simulink model "c63_cylinder_adiabatic_ref"  (R2026a)
settings: Solver=FixedStepDiscrete  StopTime=0  FixedStep=1e-4
model workspace (MAT data in the model file):
  S12_C63_BoreM = Simulink.Parameter
  S12_C63_BoreM.Value = 0.1022
  S12_C63_BoreM.Complexity = 'real'
  S12_C63_BoreM.Dimensions = [1 1]
  S12_C63_BoreM.Description = 'Grade A: Mercedes-Benz Public Archive M156.985 bore'
  S12_C63_BoreM.DataType = 'auto'
  S12_C63_BoreM.DocUnits = 'm'
  S12_C63_CompressionRatio = Simulink.Parameter
  S12_C63_CompressionRatio.Value = 11.3
  S12_C63_CompressionRatio.Complexity = 'real'
  S12_C63_CompressionRatio.Dimensions = [1 1]
  S12_C63_CompressionRatio.Description = 'Grade A: Mercedes-Benz Public Archive M156.985 compression ratio'
  S12_C63_CompressionRatio.DataType = 'auto'
  S12_C63_RodLengthM = Simulink.Parameter
  S12_C63_RodLengthM.Value = 0.1455
  S12_C63_RodLengthM.Complexity = 'real'
  S12_C63_RodLengthM.Dimensions = [1 1]
  S12_C63_RodLengthM.Description = 'Grade D identification initial value; not an OEM-fixed M156 dimension'
  S12_C63_RodLengthM.DataType = 'auto'
  S12_C63_RodLengthM.Min = 0.14
  S12_C63_RodLengthM.Max = 0.155
  S12_C63_RodLengthM.DocUnits = 'm'
  S12_C63_StrokeM = Simulink.Parameter
  S12_C63_StrokeM.Value = 0.0946
  S12_C63_StrokeM.Complexity = 'real'
  S12_C63_StrokeM.Dimensions = [1 1]
  S12_C63_StrokeM.Description = 'Grade A: Mercedes-Benz Public Archive M156.985 stroke'
  S12_C63_StrokeM.DataType = 'auto'
  S12_C63_StrokeM.DocUnits = 'm'
  S12_CrankAngleDeg = Simulink.Parameter
  S12_CrankAngleDeg.Value = 0
  S12_CrankAngleDeg.Complexity = 'real'
  S12_CrankAngleDeg.Dimensions = [1 1]
  S12_CrankAngleDeg.Description = 'Reference crank angle input; SimulationInput overrides this value during tests'
  S12_CrankAngleDeg.DataType = 'auto'
  S12_CrankAngleDeg.Min = 0
  S12_CrankAngleDeg.Max = 720
  S12_CrankAngleDeg.DocUnits = 'deg'
  S12_ReferenceGamma = Simulink.Parameter
  S12_ReferenceGamma.Value = 1.35
  S12_ReferenceGamma.Complexity = 'real'
  S12_ReferenceGamma.Dimensions = [1 1]
  S12_ReferenceGamma.Description = 'Reference constant gamma for analytic test only; S12 combustion uses temperature-dependent properties'
  S12_ReferenceGamma.DataType = 'auto'
  S12_ReferenceGamma.Min = 1.25
  S12_ReferenceGamma.Max = 1.4
  S12_ReferencePressurePa = Simulink.Parameter
  S12_ReferencePressurePa.Value = 101325
  S12_ReferencePressurePa.Complexity = 'real'
  S12_ReferencePressurePa.Dimensions = [1 1]
  S12_ReferencePressurePa.Description = 'Reference ambient pressure for analytic adiabatic test'
  S12_ReferencePressurePa.DataType = 'auto'
  S12_ReferencePressurePa.DocUnits = 'Pa'
settings Model: Creator=Jovi  LastModifiedBy=Jovi

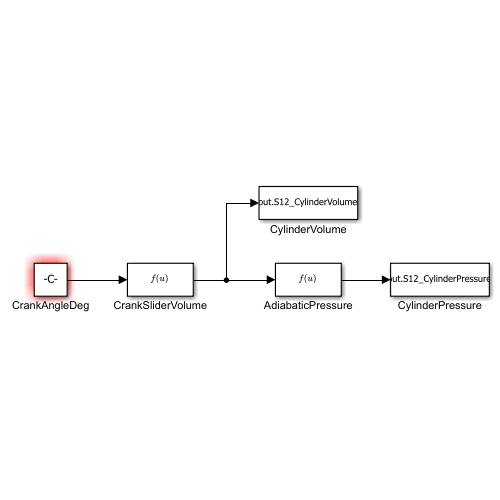
[thumbnail: Simulink's stored preview of the top-level diagram]
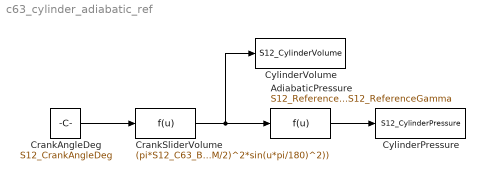
== system c63_cylinder_adiabatic_ref ==
  AdiabaticPressure : Fcn  Expr=S12_ReferencePressurePa*(((pi*S12_C63_BoreM^2*S12_C63_StrokeM/4)/(S12_C63_CompressionRatio-1) + pi*S12_C63_BoreM^2*S12_C63_StrokeM/4)/u)^S12_ReferenceGamma
  CrankAngleDeg : Constant  Value=S12_CrankAngleDeg
  CrankSliderVolume : Fcn  Expr=(pi*S12_C63_BoreM^2*S12_C63_StrokeM/4)/(S12_C63_CompressionRatio-1) + (pi*S12_C63_BoreM^2/4)*((S12_C63_StrokeM/2)*(1-cos(u*pi/180)) + S12_C63_RodLengthM - sqrt(S12_C63_RodLengthM^2 - (S12_C63_StrokeM/2)^2*sin(u*pi/180)^2))
  CylinderPressure : ToWorkspace  VariableName=S12_CylinderPressure
  CylinderVolume : ToWorkspace  VariableName=S12_CylinderVolume
  wires:
  AdiabaticPressure/1 -> CylinderPressure/1
  CrankSliderVolume/1 -> AdiabaticPressure/1, CylinderVolume/1
  CrankAngleDeg/1 -> CrankSliderVolume/1
